simulink library "qss_tb_library"  (Simulink 6.3)
undefined symbols (not defined in the file): c_BT_E1, c_BT_E2, c_BT_E3, c_BT_E4, c_BT_L1, c_BT_L2, c_BT_L3, c_BT_L4, cc_done, delta_h_C_air, dw_GG_c, eta_EG_map, eta_EM_map, g, h, H_o_m, H_u, I_BT_max, i_FC_in, i_FC_max, k1, k2, k3, k4, k_cs, M_air, manual_gearbox, P_CVT_opt, Q_BT_0, Q_BT_IC, Q_BT_min, Q_SC_IC, r_wheel, rho, rho_f, t_c, T_CE_max, T_EG_c, T_EG_max, T_EM_max, U_BT_0, V_CE_map, V_FC_out, w_CE_max, w_CE_upper, w_CVT_opt, w_EG_row, w_EG_upper, w_EM_row, w_EM_upper, w_GG_c
(part 1 of 2)
settings Model: Creator=buehli  LastModifiedBy=mo  ExtModeAutoUpdateStatusClock=off

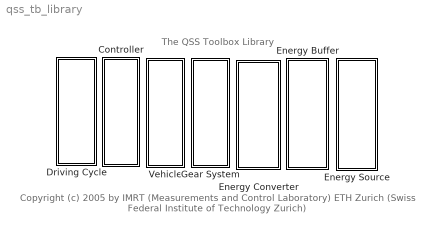
== system qss_tb_library ==
  note: Copyright (c) 2005 by IMRT (Measurements and Control Laboratory)
      | ETH Zurich (Swiss Federal Institute of Technology Zurich)
  note: The QSS Toolbox Library
  Controller : Subsystem  Orientation=up
      mask Display: disp('Controller')
  Driving Cycle : Subsystem  Orientation=up
      mask Display: disp('Driving Cycle')
  Energy Buffer : Subsystem  Orientation=up
      mask Display: disp('Energy Buffer')
  Energy Converter : Subsystem  Orientation=up
      mask Display: disp('Energy Converter')
  Energy Source : Subsystem  Orientation=up
      mask Display: disp('Energy Source')
  Gear System : Subsystem  Orientation=up
      mask Display: disp('Gear System')
  Vehicle : Subsystem  Orientation=up
      mask Display: disp('Vehicle')

== system qss_tb_library/Controller ==
  Battery Controller : Subsystem  AncestorBlock=qss_tb_library/Controller/Battery Controller  mask(Battery Controller){}
      mask help:
      | Control strategy (very primitive):
      | ========================
      | As soon as battery charge drops below level Q_BT_min, the CE/Generator
      | are started and operated at given load/speed for a fixed time period.
      | This time has been selected to guarantee the same battery level at the
      | end of the cycle.
      mask init:
      | init_BT_ctrl;
  CVT Controller : Subsystem  Tag=cvt controller  mask(CVT Controller){j_CVT_min=3, j_CVT_max=15, w_wheel_min=3, w_CVT_idle=100, w_CVT_upper=300}
      mask prompts: j_CVT_min "Lower gear ratio limit [-]"; j_CVT_max "Upper gear ratio limit [-]"; w_wheel_min "Minimum wheel speed [rad/s]"; w_CVT_idle "CVT idle speed [rad/s]"; w_CVT_upper "Maximum CVT speed [rad/s]"
      mask help:
      | This block calculates the optimum gear ratio and its change during one integration step for a CVT.
      |
      | Input:
      | =====
      | 	v		Speed [m/s]
      | 	dv		Acceleration [m/s^2]
      |
      | Output:
      | ======
      | 	v_delay		Speed one step delayed [m/s]
      | 	dv_delay	Acceleration one step delayed [m/s^2]
      | 	j_CVT		Gear ratio [-]
      | 	dj_CVT		Change of gear ratio [1/s]
      mask init:
      | init_CVT_ctrl;
  Control Unit (empty template) : Subsystem  Tag=control unit
      mask Type: Control Unit
      mask Description:
      | This block gives the user the opportunity to design his/her own control unit.
      | 
      | The user can define the inputs and outputs  by himself/herself.

== system qss_tb_library/Driving Cycle ==
  Driving Cycle : Subsystem  Tag=cycle  mask(Driving Cycle){cyclenr=Europe: NEDC, stepsize=1, autostop=on}
      mask prompts: cyclenr "Choose a cycle"; stepsize "Step size [s]"; autostop "Enable automatic simulation stop"
      mask help:
      | This block loads the cycle data such as time, speed, acceleration and gear number,  from the specified data file and makes it available on the output of the cycle block.
      |
      | Output:
      | ======
      | 	v	Speed [m/s]
      | 	dv	Acceleration [m/s^2]
      | 	i	Gear number [-]
      | 	x_tot	Total distance [m]
      |
      | Tip:
      | ===
      | Probably you don't need the gear number "i". If so you can terminate
      | it with a "Terminator" out of the "Simulink Library/Connections."
      |
      | Step size:
      | ========
      | Default value is 1. Don't change it, unless you are familiar with the programs of the QSS TB.
      |
      | Enable automatic simulation stop:
      | ===========================
      | Stops the simulation automatically at the end of the cycle.
      | Be careful: If you have a component in your model that has to run after the cycle has finished, e.g. a battery to charge, remove the mark!
      mask init:
      | init_driving_cycle;
      mask StyleString: popup(Europe: ECE manual|Europe: ECE R15 spez|Europe: ECE R15|Europe: EUDC|Europe: EUDC manual|Europe: City|Europe: City manual|Europe: NEDC|Europe: NEDC manual|Japan:  10-15-Mode|Japan:  10-Mode|Japan:  10-Mode-3|Japan:  11-Mode|Japan:  11-Mode-4|Japan:  15-Mode|USA:    City-I|USA:    City-II|USA:    FTP-75|USA:    FTP-Highway),edit,checkbox
      mask Display: plot(T_zplot, V_zplot);

== system qss_tb_library/Energy Buffer ==
  Battery : Subsystem  Tag=battery  mask(Battery){I_0=100, Q_BT_IC_rel=27.78, t_ch=20}
      mask prompts: I_0 "Energy capacity of battery [Ah]"; Q_BT_IC_rel "Initial charge of battery [%]"; t_ch "Current limit: minimum time to charge/discharge the battery [min]"
      mask help:
      | This block simulates a battery.
      | The resistance depends on the charge state and the charge/discharge current of the battery. The battery has an open circuit voltage of 130 V (fully charged).
      |
      | Input:
      | =====
      | 	x_tot	Total distance [m]
      | 	P_BT	Power from/to the battery [W]
      | 		P_BT < 0: battery charging
      | 		P_BT > 0: battery discharging
      |
      | Output:
      | ======
      | 	Q_BT	Current charge of the battery [C]
      | 	V_BT	Energy consumption [kWh/100 km]
      mask init:
      | init_BT;
  Supercapacitor : Subsystem  Tag=supercap  mask(Supercapacitor){C_SC=8, R_SC=0.72, U_SC_max=225, P_SC_max=17500, Q_SC_IC_rel=95, N_SC=6}
      mask prompts: C_SC "Capacity of each supercap [F]"; R_SC "Internal resistance of each supercap [Ohm]"; U_SC_max "Maximum voltage of each supercap  [V]"; P_SC_max "Maximum power of each supercap [W]"; Q_SC_IC_rel "Initial charge of each supercap [%]"; N_SC "Number of supercaps (parallel connection) [-]"
      mask help:
      | The supercap is a fast electric energy buffer.
      |
      | Input:
      | =====
      | 	P_SC	Power to/from the supercap [W]
      | 		P_SC < 0: SC charging
      | 		P_SC > 0: SC discharging
      |
      | Output:
      | ======
      | 	U_SC	Voltage of the supercap [V]
      mask init:
      | init_SC;

== system qss_tb_library/Energy Converter ==
  Combustion Engine (Willans-approximation) : Subsystem  Tag=combustion engine  AncestorBlock=qss_lib/Energy Converter/combustion engine  mask(Combustion Engine (based on Willans approximation)){engine_type=Otto, V_d=0.708, theta_CE=0.05, S=50, B=45, w_CE_idle=105, P_CE_idle=2600, P_aux=300, e=0.46, PI=2, p_me0g=1, ENABLE_FUEL_CUTOFF=on, T_CE_cutoff=5, P_CE_cutoff=0}
      mask prompts: engine_type "Engine type"; V_d "Displacement [l]"; theta_CE "Engine inertia [kg*m^2]"; S "Stroke [mm]"; B "Bore diameter [mm]"; w_CE_idle "Engine speed at idle [rad/s]"; P_CE_idle "Engine power at idle [W]"; P_aux "Power required by auxiliaries  [W]"; e "1. Willans parameter: Engine internal thermodynamic efficiency [-]"; PI "2. Willans parameter: Maximum boost ratio [-]"; p_me0g "3. Willans parameter: Gas exchange losses [bar]"; ENABLE_FUEL_CUTOFF "Enable fuel cutoff"; T_CE_cutoff "Engine torque at fuel cutoff [Nm]"; P_CE_cutoff "Power at fuel cutoff [W]"
      mask help:
      | This block simulates the behaviour of a combustion engine. The block is based on the Willans approximation with friction part based on the ETH model.
      |
      | Input:
      | =====
      | 	w_gear		Speed of the fly wheel [rad/s]
      | 	dw_gear	Acceleration of the fly wheel [rad/s^2]
      | 	T_gear		Torque on the fly wheel [Nm]
      |
      | Output:
      | ======
      | 	P_CE		Power produced by the combustion engine [W]
      mask init:
      | init_CE_willans;
      mask StyleString: popup(Otto|Diesel),edit,edit,edit,edit,edit,edit,edit,edit,edit,edit,checkbox,edit,edit
  Combustion Engine (consumption map) : Subsystem  Tag=combustion engine  AncestorBlock=QSS_TB_lib/Energy Converter/Combustion Engine  mask(Combustion Engine (based on consumption map)){engine_type=Otto, V_d=0.708, scale_CE=1, theta_CE=0.05, w_CE_idle=105, P_CE_idle=2600, P_aux=300, ENABLE_FUEL_CUTOFF=on, T_CE_cutoff=5, P_CE_cutoff=0}
      mask prompts: engine_type "Engine type"; V_d "Displacement [l]"; scale_CE "Engine scaling factor [-]"; theta_CE "Engine inertia [kg*m^2]"; w_CE_idle "Engine speed at idle [rad/s]"; P_CE_idle "Engine power at idle [W]"; P_aux "Power required by auxiliaries [W]"; ENABLE_FUEL_CUTOFF "Enable fuel cutoff"; T_CE_cutoff "Engine torque at fuel cutoff [Nm]"; P_CE_cutoff "Power at fuel cutoff [W]"
      mask help:
      | This block simulates the behaviour of a combustion engine. The block is based on a consumption map.
      |
      | Input:
      | =====
      | 	w_gear		Speed of the fly wheel [rad/s]
      | 	dw_gear	Acceleration of the fly wheel [rad/s^2]
      | 	T_gear		Torque on the fly wheel [Nm]
      |
      | Output:
      | ======
      | 	P_CE		Power produced by the combustion engine [W]
      mask init:
      | init_CE_map;
      mask StyleString: popup(Otto|Diesel),edit,edit,edit,edit,edit,edit,checkbox,edit,edit
  Electric Generator : Subsystem  AncestorBlock=QSS_TB_lib/Energy Converter/Electric Motor  mask(Electric Generator){scale_EG=1}
      mask prompts: scale_EG "Generator scaling factor [-]"
      mask help:
      | This block simulates the behaviour of an electric generator. The block is based on an efficiency map.
      |
      | Input:
      | =====
      | 	w_gear		Speed of the fly wheel [rad/s]
      | 	T_gear		Torque on the fly wheel [Nm]
      |
      | Output:
      | ======
      | 	P_EG		Power of the electric generator [W]
      mask init:
      | init_EG;
  Electric Motor : Subsystem  mask(Electric Motor){scale_EM=1, theta_EM=0.1, P_aux=0}
      mask prompts: scale_EM "Motor scaling factor [-]"; theta_EM "Motor inertia [kg*m2]"; P_aux "Power required by auxiliaries [W]"
      mask help:
      | This block simulates the behaviour of an electric motor. The block is based on an efficiency map.
      |
      | Input:
      | =====
      | 	w_gear		Speed of the fly wheel [rad/s]
      | 	dw_gear	Acceleration of the fly wheel [rad/s^2]
      | 	T_gear		Torque on the fly wheel [Nm]
      |
      | Output:
      | ======
      | 	P_EM		Power produced by the electric motor [W]
      mask init:
      | init_EM;
  Fuel Cell : Subsystem  Tag=fuelcell  mask(Fuel Cell){N_FC=880, A_FC=190 * 1e4, V_th=1.2, P_FC_idle=2000, eta_EM_C=0.75, eta_C=0.7, pi_C=1.3, T_air=25, l_air=1.5}
      mask prompts: N_FC "Number of fuel cells per stack (series connection) [-]"; A_FC "Size of fuel cell [m^2]"; V_th "Theoretical fuel cell voltage [V]"; P_FC_idle "Idle power [W]"; eta_EM_C "E-motor for air compressor efficiency [-]"; eta_C "Air compressor efficiency [-]"; pi_C "Air compression ratio [-]"; T_air "Air temperature [°C]"; l_air "Air to fuel ratio [-]"
      mask help:
      | This block simulates a fuel cell and converts fuel into electric energy.
      |
      | Input:
      | =====
      | 	P_in		Power required by the fuel cell [W]
      |
      | Output:
      | ======
      | 	P_FC		Power produced by the fuel cell [W]
      mask init:
      | init_FC;

== system qss_tb_library/Energy Source ==
  Display : Display
  Tank : Subsystem  Tag=tank  mask(Tank){fuel=Gasoline, flag_cold_start=on}
      mask prompts: flag_cold_start "Include cold start losses"
      mask help:
      | This block integrates the power (the fuel mass flow) required by the combustion engine or the fuel cell and calculates the energy consumption in liter/100 km.
      |
      | Input:
      | =====
      | 	P_fuel	Power (fuel mass flow) required [W]
      | 	x_tot	Total distance [m]
      |
      | Output:
      | ======
      | 	V	Fuel consumption [liter/100 km]
      mask init:
      | init_tank;
      mask StyleString: popup(Gasoline|Diesel|Hydrogen),checkbox
  wires:
  Tank/1(liter/100 km) -> Display/1

== system qss_tb_library/Gear System ==
  Continuously Variable Transmission : Subsystem  Tag=cvt  mask(CVT){e_CVT=0.97, P_CVT0=400, w_wheel_min=3}
      mask prompts: e_CVT "Efficiency [-]"; P_CVT0 "Idling losses (friction) [W]"; w_wheel_min "Minimum wheel speed beyond which losses are generated [rad/s]"
      mask help:
      | This block simulates a CVT transmission.
      |
      | Input:
      | =====
      | 	w_wheel	Speed of the wheel [rad/s]
      | 	dw_wheel	Acceleration of the wheel [rad/s^2],
      | 	T_wheel	Torque on the wheel [Nm]
      | 	j_CVT		Gear ratio [-]
      | 	dj_CVT		Change of gear ratio [1/s]
      |
      | Output:
      | ======
      | 	w_CVT		Speed of the fly wheel [rad/s]
      | 	dw_CVT	Acceleration of the fly wheel [rad/s^2]
      | 	T_CVT		Torque on the fly wheel [Nm]
      mask init:
      | init_CVT;
  Manual Gear Box : Subsystem  Tag=transmission  mask(Manual Gear Box){i_1=15.174, i_2=8.338, i_3=5.378, i_4=3.937, i_5=2.748, i_diff=1, e_GT=0.98, P_GT0=300, w_wheel_min=1}
      mask prompts: i_1 "1. gear [-]"; i_2 "2. gear [-]"; i_3 "3. gear [-]"; i_4 "4. gear [-]"; i_5 "5. gear [-]"; i_diff "Differential gear [-]"; e_GT "Efficiency [-]"; P_GT0 "Idling losses (friction) [W]"; w_wheel_min "Minimum wheel speed beyond which losses are generated [rad/s]"
      mask help:
      | This block simulates a manual gear box.
      |
      | Input:
      | =====
      | 	w_wheel	Speed of the wheel [rad/s]
      | 	dw_wheel	Acceleration of the wheel [rad/s^2],
      | 	T_wheel	Torque on the wheel [Nm]
      | 	i		Gear number [-]
      |
      | Output:
      | ======
      | 	w_MGB		Speed of the fly wheel [rad/s]
      | 	dw_MGB	Acceleration of the fly wheel [rad/s^2]
      | 	T_MGB		Torque on the fly wheel [Nm]
      mask init:
      | init_MGB;
  Simple Transmission : Subsystem  Tag=simple transmission  mask(Simple Transmission){gear_ratio=3, e_GT=0.98, P_GT0=50, w_wheel_min=1}
      mask prompts: gear_ratio "Gear ratio [-]"; e_GT "Efficiency [-]"; P_GT0 "Idling losses (friction) [W]"; w_wheel_min "Minimum wheel speed beyond which losses are generated [rad/s]"
      mask help:
      | This block simulates a transmission with a fixed gear ratio.
      |
      | Input:
      | =====
      | 	w_wheel	Speed of the wheel [rad/s]
      | 	dw_wheel	Acceleration of the wheel [rad/s^2]
      | 	T_wheel	Torque on the wheel [Nm]
      |
      | Output:
      | ======
      | 	w_trans		Speed of the fly wheel [rad/s]
      | 	dw_trans	Acceleration of the fly wheel [rad/s^2]
      | 	T_trans		Torque on the fly wheel [Nm]
      mask init:
      | init_transmission;

== system qss_tb_library/Vehicle ==
  Vehicle : Subsystem  Tag=vehicle  mask(Vehicle){m_f=750, mt2m_f=5, A_f=1.8, d_wheel=0.5, cw=0.22, mu=0.008}
      mask prompts: m_f "Total mass of the vehicle [kg]"; mt2m_f "Rotating mass [%]"; A_f "Vehicle cross section [m^2]"; d_wheel "Wheel diameter [m]"; cw "Drag coefficient [-]"; mu "Rolling friction coefficient [-]"
      mask help:
      | This block computes the power required from the vehicle.
      |
      | Input:
      | =====
      | 	v		Speed [m/s]
      | 	dv		Acceleration [m/s^2]
      |
      | Output:
      | ======
      | 	w_wheel	Speed of the wheel [rad/s]
      | 	dw_wheel	Acceleration of the wheel [rad/s^2]
      | 	T_wheel	Torque on the wheel [Nm]
      mask init:
      | init_vehicle;

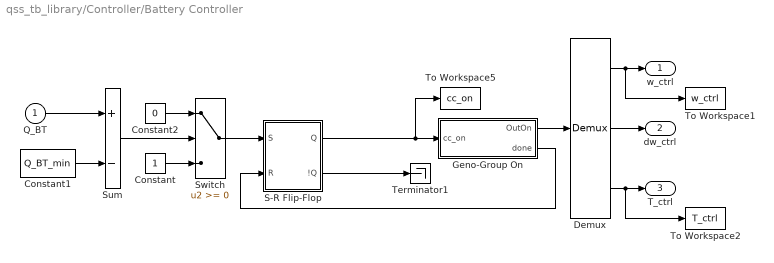
== system qss_tb_library/Controller/Battery Controller ==
  Q_BT : Inport
  Constant : Constant  OutDataTypeMode=boolean
  Constant1 : Constant  Value=Q_BT_min
  Constant2 : Constant  Value=0  OutDataTypeMode=boolean
  Demux : Demux  Outputs=3
  Geno-Group On : Subsystem
  S-R Flip-Flop : Subsystem
  Sum : Sum  Inputs=+-  SaturateOnIntegerOverflow=on  InputSameDT=on
  Switch : Switch  SaturateOnIntegerOverflow=on  InputSameDT=on
  Terminator1 : Terminator
  To Workspace1 : ToWorkspace  VariableName=w_ctrl  SampleTime=-1  SaveFormat=Array
  To Workspace2 : ToWorkspace  VariableName=T_ctrl  SampleTime=-1  SaveFormat=Array
  To Workspace5 : ToWorkspace  VariableName=cc_on  SampleTime=-1  SaveFormat=Array
  w_ctrl : Outport  InitialOutput=0
  dw_ctrl : Outport  Port=2  InitialOutput=0
  T_ctrl : Outport  Port=3  InitialOutput=0
  wires:
  S-R Flip-Flop/1(Q) -> To Workspace5/1, Geno-Group On/1(cc_on)
  Switch/1 -> S-R Flip-Flop/1(S)
  S-R Flip-Flop/2(!Q) -> Terminator1/1
  Geno-Group On/1(OutOn) -> Demux/1
  Demux/3 -> To Workspace2/1, T_ctrl/1
  Demux/2 -> dw_ctrl/1
  Demux/1 -> To Workspace1/1, w_ctrl/1
  Geno-Group On/2(done) -> S-R Flip-Flop/2(R)
  Q_BT/1 -> Sum/1
  Sum/1 -> Switch/2
  Constant2/1 -> Switch/1
  Constant/1 -> Switch/3
  Constant1/1 -> Sum/2

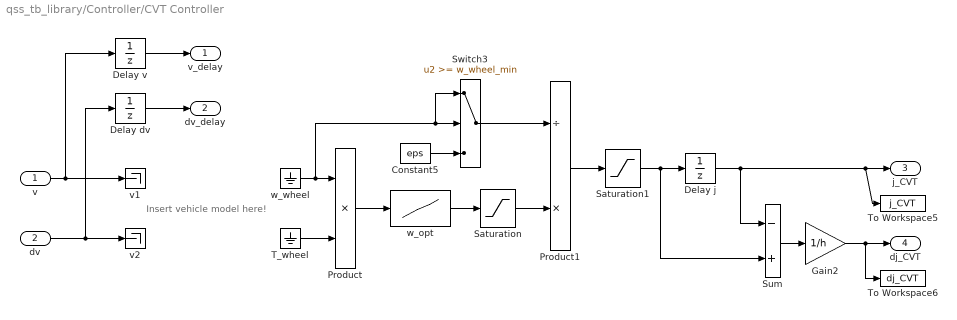
== system qss_tb_library/Controller/CVT Controller ==
  note: Insert vehicle
      | model here!
  v : Inport
  dv : Inport  Port=2
  Constant5 : Constant  Value=eps
  Delay dv : UnitDelay  SampleTime=h
  Delay j : UnitDelay  X0=j_CVT_min  SampleTime=h
  Delay v : UnitDelay  SampleTime=h
  Gain2 : Gain  Gain=1/h  SaturateOnIntegerOverflow=on
  Product : Product  SaturateOnIntegerOverflow=on  RndMeth=Zero  InputSameDT=on
  Product1 : Product  Inputs=/*  SaturateOnIntegerOverflow=on  RndMeth=Zero  InputSameDT=on
  Saturation : Saturate  UpperLimit=w_CVT_upper  LowerLimit=w_CVT_idle
  Saturation1 : Saturate  UpperLimit=j_CVT_max  LowerLimit=j_CVT_min
  Sum : Sum  Inputs=-+  SaturateOnIntegerOverflow=on  InputSameDT=on
  Switch3 : Switch  Threshold=w_wheel_min  SaturateOnIntegerOverflow=on  InputSameDT=on
  T_wheel : Ground
  To Workspace5 : ToWorkspace  VariableName=j_CVT  SampleTime=-1  SaveFormat=Array
  To Workspace6 : ToWorkspace  VariableName=dj_CVT  SampleTime=-1  SaveFormat=Array
  v1 : Terminator
  v2 : Terminator
  w_opt : Lookup  InputValues=P_CVT_opt  OutputValues=w_CVT_opt  SaturateOnIntegerOverflow=on
  w_wheel : Ground
  v_delay : Outport  InitialOutput=0
  dv_delay : Outport  Port=2  InitialOutput=0
  j_CVT : Outport  Port=3  InitialOutput=0
  dj_CVT : Outport  Port=4  InitialOutput=0
  wires:
  Gain2/1 -> To Workspace6/1, dj_CVT/1
  T_wheel/1 -> Product/2
  Product1/1 -> Saturation1/1
  Saturation/1 -> Product1/2
  w_wheel/1 -> Switch3/2, Switch3/1, Product/1
  Constant5/1 -> Switch3/3
  dv/1 -> Delay dv/1, v2/1
  v/1 -> Delay v/1, v1/1
  Delay dv/1 -> dv_delay/1
  Switch3/1 -> Product1/1
  Delay j/1 -> To Workspace5/1, j_CVT/1, Sum/1
  Saturation1/1 -> Delay j/1, Sum/2
  Product/1 -> w_opt/1
  w_opt/1 -> Saturation/1
  Delay v/1 -> v_delay/1
  Sum/1 -> Gain2/1

== system qss_tb_library/Controller/Control Unit (empty template) ==
  note: Control Unit: custom designed
  y 1 : Inport
  y p : Inport  Port=2
  Ground : Ground
  Ground1 : Ground
  Terminator : Terminator
  Terminator1 : Terminator
  u 1 : Outport  InitialOutput=0
  u m : Outport  Port=2  InitialOutput=0
  wires:
  Ground/1 -> u 1/1
  Ground1/1 -> u m/1
  y 1/1 -> Terminator/1
  y p/1 -> Terminator1/1

== system qss_tb_library/Driving Cycle/Driving Cycle ==
  note: Speed
  Clock : Clock
      settings: Decimation=10
  Cycle data : FromWorkspace  VariableName=[T_z, V_z, D_z, G_z]  SampleTime=h
  Demux : Demux  Outputs=3
  Differentiation : Subsystem
  Integration : Subsystem
  Terminator : Terminator
  Time : Display
  To Workspace1 : ToWorkspace  VariableName=t  SampleTime=-1  SaveFormat=Array
  To Workspace2 : ToWorkspace  VariableName=x_tot  SampleTime=-1  SaveFormat=Array
  To Workspace4 : ToWorkspace  VariableName=dv  SampleTime=-1  SaveFormat=Array
  To Workspace5 : ToWorkspace  VariableName=v  SampleTime=-1  SaveFormat=Array
  To Workspace6 : ToWorkspace  VariableName=i  SampleTime=-1  SaveFormat=Array
  v : Outport  InitialOutput=0
  dv : Outport  Port=2  InitialOutput=0
  i : Outport  Port=3  InitialOutput=0
  x_tot : Outport  Port=4  InitialOutput=0
  wires:
  Cycle data/1 -> Demux/1
  Differentiation/1(D_z) -> To Workspace4/1, dv/1
  Demux/2 -> Terminator/1
  Demux/1 -> Integration/1(V_z), v/1, To Workspace5/1, Differentiation/1(V_z)
  Integration/1(x_tot) -> x_tot/1, To Workspace2/1
  Demux/3 -> i/1, To Workspace6/1  "Gear ratio"
  Clock/1 -> Time/1, To Workspace1/1

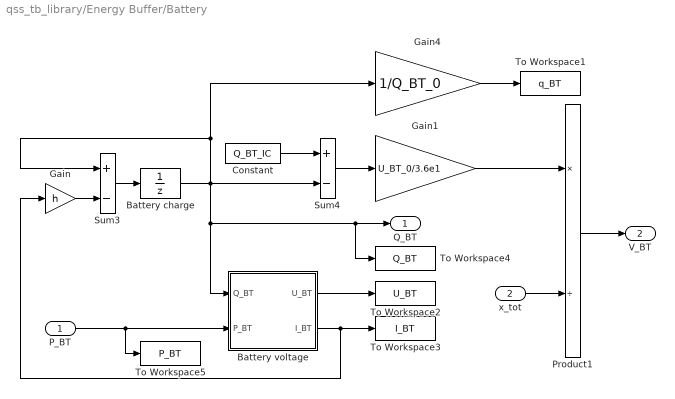
== system qss_tb_library/Energy Buffer/Battery ==
  P_BT : Inport
  x_tot : Inport  Port=2
  Battery charge : UnitDelay  X0=Q_BT_IC  SampleTime=h
  Battery voltage : Subsystem
  Constant : Constant  Value=Q_BT_IC
  Gain : Gain  Gain=h  SaturateOnIntegerOverflow=on
  Gain1 : Gain  Gain=U_BT_0/3.6e1  SaturateOnIntegerOverflow=on
  Gain4 : Gain  Gain=1/Q_BT_0  SaturateOnIntegerOverflow=on
  Product1 : Product  Inputs=*/  SaturateOnIntegerOverflow=on  RndMeth=Zero  InputSameDT=on
  Sum3 : Sum  Inputs=+-  SaturateOnIntegerOverflow=on  InputSameDT=on
  Sum4 : Sum  Inputs=+-  SaturateOnIntegerOverflow=on  InputSameDT=on
  To Workspace1 : ToWorkspace  VariableName=q_BT  SampleTime=-1  SaveFormat=Array
  To Workspace2 : ToWorkspace  VariableName=U_BT  SampleTime=-1  SaveFormat=Array
  To Workspace3 : ToWorkspace  VariableName=I_BT  SampleTime=-1  SaveFormat=Array
  To Workspace4 : ToWorkspace  VariableName=Q_BT  SampleTime=-1  SaveFormat=Array
  To Workspace5 : ToWorkspace  VariableName=P_BT  SampleTime=-1  SaveFormat=Array
  Q_BT : Outport  InitialOutput=0
  V_BT : Outport  Port=2  InitialOutput=0
  wires:
  Battery voltage/2(I_BT) -> Gain/1, To Workspace3/1
  Constant/1 -> Sum4/1
  Sum3/1 -> Battery charge/1
  Gain/1 -> Sum3/2
  Battery charge/1 -> Sum3/1, Gain4/1, Sum4/2, Battery voltage/1(Q_BT), Q_BT/1, To Workspace4/1
  Battery voltage/1(U_BT) -> To Workspace2/1
  x_tot/1 -> Product1/2
  Gain1/1 -> Product1/1
  Product1/1 -> V_BT/1
  Sum4/1 -> Gain1/1
  Gain4/1 -> To Workspace1/1
  P_BT/1 -> Battery voltage/2(P_BT), To Workspace5/1

== system qss_tb_library/Energy Buffer/Supercapacitor ==
  P_SC : Inport
  Fcn : Fcn  Expr=(-u[2]/C_SC+sqrt(u[2]^2/C_SC^2-4*R_SC*u[1]))/(2*R_SC)
  Gain : Gain  Gain=1/C_SC  SaturateOnIntegerOverflow=on
  Gain1 : Gain  Orientation=left  Gain=h  SaturateOnIntegerOverflow=on
  Mux : Mux  Inputs=2
  SC charge : UnitDelay  Orientation=left  X0=Q_SC_IC  SampleTime=h
  Sum3 : Sum  Orientation=left  SaturateOnIntegerOverflow=on  InputSameDT=on
  Supervision supercap : Subsystem
  To Workspace1 : ToWorkspace  VariableName=I_SC  SampleTime=1  SaveFormat=Array
  To Workspace2 : ToWorkspace  VariableName=U_SC  SampleTime=1  SaveFormat=Array
  To Workspace3 : ToWorkspace  VariableName=Q_SC  SampleTime=1  SaveFormat=Array
  To Workspace4 : ToWorkspace  VariableName=P_SC  SampleTime=1  SaveFormat=Array
  U_SC : Outport  InitialOutput=0
  wires:
  P_SC/1 -> Supervision supercap/2(P_SC), Mux/1, To Workspace4/1
  Gain/1 -> To Workspace2/1, U_SC/1
  Fcn/1 -> To Workspace1/1, Gain1/1
  SC charge/1 -> To Workspace3/1, Supervision supercap/1(Q_SC), Mux/2, Gain/1, Sum3/2
  Sum3/1 -> SC charge/1
  Mux/1 -> Fcn/1
  Gain1/1 -> Sum3/1

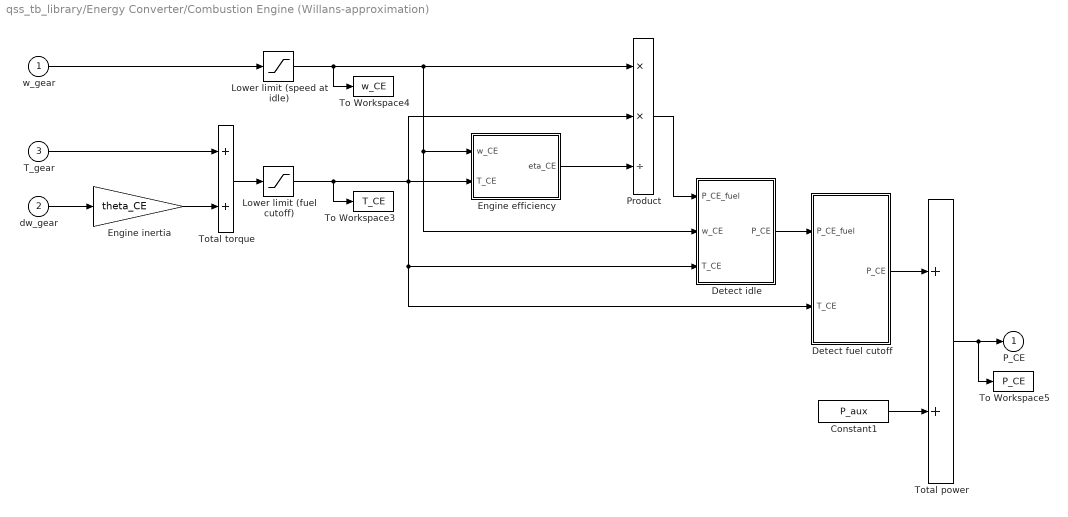
== system qss_tb_library/Energy Converter/Combustion Engine (Willans-approximation) ==
  w_gear : Inport
  dw_gear : Inport  Port=2
  T_gear : Inport  Port=3
  Constant1 : Constant  Value=P_aux
  Detect fuel cutoff : Subsystem  AncestorBlock=|
      | qss_tb_library/Energy Converter/Combustion Engine
      | (consumption map)/Detect fuel cutoff
  Detect idle : Subsystem
  Engine efficiency : Subsystem
  Engine inertia : Gain  Gain=theta_CE  SaturateOnIntegerOverflow=on
  Lower limit (fuel cutoff) : Saturate  UpperLimit=inf  LowerLimit=T_CE_cutoff
  Lower limit (speed at idle) : Saturate  UpperLimit=inf  LowerLimit=w_CE_idle
  Product : Product  Inputs=**/  SaturateOnIntegerOverflow=on  RndMeth=Zero  InputSameDT=on
  To Workspace3 : ToWorkspace  VariableName=T_CE  SampleTime=-1  SaveFormat=Array
  To Workspace4 : ToWorkspace  VariableName=w_CE  SampleTime=-1  SaveFormat=Array
  To Workspace5 : ToWorkspace  VariableName=P_CE  SampleTime=-1  SaveFormat=Array
  Total power : Sum  SaturateOnIntegerOverflow=on  InputSameDT=on
  Total torque : Sum  SaturateOnIntegerOverflow=on  InputSameDT=on
  P_CE : Outport  InitialOutput=0
  wires:
  Engine efficiency/1(eta_CE) -> Product/3
  T_gear/1 -> Total torque/1
  dw_gear/1 -> Engine inertia/1
  Total torque/1 -> Lower limit (fuel cutoff)/1
  Engine inertia/1 -> Total torque/2
  Lower limit (fuel cutoff)/1 -> Detect idle/3(T_CE), Detect fuel cutoff/2(T_CE), Engine efficiency/2(T_CE), Product/2, To Workspace3/1
  Lower limit (speed at idle)/1 -> To Workspace4/1, Engine efficiency/1(w_CE), Detect idle/2(w_CE), Product/1
  w_gear/1 -> Lower limit (speed at idle)/1
  Product/1 -> Detect idle/1(P_CE_fuel)
  Detect idle/1(P_CE) -> Detect fuel cutoff/1(P_CE_fuel)
  Detect fuel cutoff/1(P_CE) -> Total power/1
  Total power/1 -> P_CE/1, To Workspace5/1
  Constant1/1 -> Total power/2

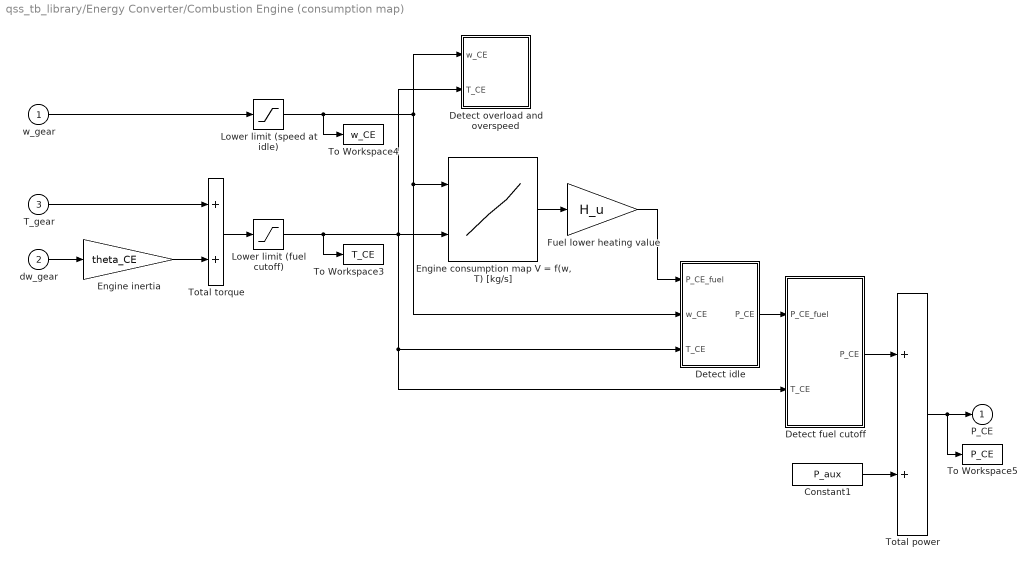
== system qss_tb_library/Energy Converter/Combustion Engine (consumption map) ==
  w_gear : Inport
  dw_gear : Inport  Port=2
  T_gear : Inport  Port=3
  Constant1 : Constant  Value=P_aux
  Detect fuel cutoff : Subsystem
  Detect idle : Subsystem
  Detect overload and overspeed : Subsystem
  "Engine consumption map V = f(w, T) [kg/s]" : Lookup2D  RowIndex=w_CE_row  ColumnIndex=T_CE_col  OutputValues=V_CE_map
  Engine inertia : Gain  Gain=theta_CE  SaturateOnIntegerOverflow=on
  Fuel lower heating value : Gain  Gain=H_u  SaturateOnIntegerOverflow=on
  Lower limit (fuel cutoff) : Saturate  UpperLimit=inf  LowerLimit=T_CE_cutoff
  Lower limit (speed at idle) : Saturate  UpperLimit=inf  LowerLimit=w_CE_idle
  To Workspace3 : ToWorkspace  VariableName=T_CE  SampleTime=-1  SaveFormat=Array
  To Workspace4 : ToWorkspace  VariableName=w_CE  SampleTime=-1  SaveFormat=Array
  To Workspace5 : ToWorkspace  VariableName=P_CE  SampleTime=-1  SaveFormat=Array
  Total power : Sum  SaturateOnIntegerOverflow=on  InputSameDT=on
  Total torque : Sum  SaturateOnIntegerOverflow=on  InputSameDT=on
  P_CE : Outport  InitialOutput=0
  wires:
  T_gear/1 -> Total torque/1
  dw_gear/1 -> Engine inertia/1
  Total torque/1 -> Lower limit (fuel cutoff)/1
  Engine inertia/1 -> Total torque/2
  Lower limit (speed at idle)/1 -> Detect overload and overspeed/1(w_CE), Detect idle/2(w_CE), "Engine consumption map V = f(w, T) [kg/s]"/1, To Workspace4/1
  w_gear/1 -> Lower limit (speed at idle)/1
  Fuel lower heating value/1 -> Detect idle/1(P_CE_fuel)
  Detect idle/1(P_CE) -> Detect fuel cutoff/1(P_CE_fuel)
  "Engine consumption map V = f(w, T) [kg/s]"/1 -> Fuel lower heating value/1
  Detect fuel cutoff/1(P_CE) -> Total power/1
  Total power/1 -> P_CE/1, To Workspace5/1
  Constant1/1 -> Total power/2
  Lower limit (fuel cutoff)/1 -> Detect overload and overspeed/2(T_CE), "Engine consumption map V = f(w, T) [kg/s]"/2, Detect idle/3(T_CE), Detect fuel cutoff/2(T_CE), To Workspace3/1

== system qss_tb_library/Energy Converter/Electric Generator ==
  w_gear : Inport
  T_gear : Inport  Port=2
  Detect overload and overspeed : Subsystem
  "Efficiency eta = f(w, T)" : Lookup2D  RowIndex=w_EG_row  ColumnIndex=T_EG_col  OutputValues=eta_EG_map
  Product : Product  Inputs=3  SaturateOnIntegerOverflow=on  RndMeth=Zero  InputSameDT=on
  To Workspace1 : ToWorkspace  VariableName=w_EG  SampleTime=-1  SaveFormat=Array
  To Workspace2 : ToWorkspace  VariableName=T_EG  SampleTime=-1  SaveFormat=Array
  To Workspace5 : ToWorkspace  VariableName=P_EG  SampleTime=-1  SaveFormat=Array
  P_EG : Outport  InitialOutput=0
  wires:
  T_gear/1 -> Product/2, "Efficiency eta = f(w, T)"/2, Detect overload and overspeed/2(T_EG), To Workspace2/1
  "Efficiency eta = f(w, T)"/1 -> Product/1
  Product/1 -> P_EG/1, To Workspace5/1
  w_gear/1 -> Product/3, "Efficiency eta = f(w, T)"/1, Detect overload and overspeed/1(w_EG), To Workspace1/1

== system qss_tb_library/Energy Converter/Electric Motor ==
  w_gear : Inport
  dw_gear : Inport  Port=2
  T_gear : Inport  Port=3
  Constant1 : Constant  Value=P_aux
  Detect overload and overspeed : Subsystem
  "Efficiency eta = f(w, T)" : Lookup2D  RowIndex=w_EM_row  ColumnIndex=T_EM_col  OutputValues=eta_EM_map
  Gain1 : Gain  Gain=theta_EM  SaturateOnIntegerOverflow=on
  Product : Product  Inputs=3  SaturateOnIntegerOverflow=on  RndMeth=Zero  InputSameDT=on
  To Workspace1 : ToWorkspace  VariableName=w_EM  SampleTime=-1  SaveFormat=Array
  To Workspace2 : ToWorkspace  VariableName=T_EM  SampleTime=-1  SaveFormat=Array
  To Workspace5 : ToWorkspace  VariableName=P_EM  SampleTime=-1  SaveFormat=Array
  Total power : Sum  SaturateOnIntegerOverflow=on  InputSameDT=on
  Total torque : Sum  SaturateOnIntegerOverflow=on  InputSameDT=on
  P_EM : Outport  InitialOutput=0
  wires:
  w_gear/1 -> Detect overload and overspeed/1(w_EM), "Efficiency eta = f(w, T)"/1, Product/3, To Workspace1/1
  "Efficiency eta = f(w, T)"/1 -> Product/1
  dw_gear/1 -> Gain1/1
  T_gear/1 -> Total torque/2
  Gain1/1 -> Total torque/1
  Total torque/1 -> Detect overload and overspeed/2(T_EM), "Efficiency eta = f(w, T)"/2, Product/2, To Workspace2/1
  Constant1/1 -> Total power/2
  Product/1 -> Total power/1
  Total power/1 -> P_EM/1, To Workspace5/1

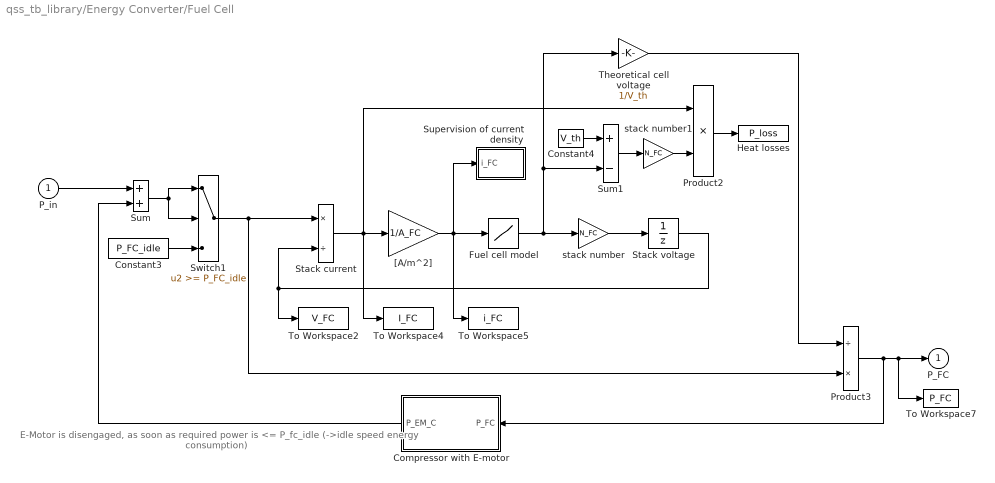
== system qss_tb_library/Energy Converter/Fuel Cell ==
  note: E-Motor is disengaged, as soon as required power
      |  is <= P_fc_idle (->idle speed energy consumption)
  P_in : Inport
  Compressor with E-motor : Subsystem  Orientation=left
  Constant3 : Constant  Value=P_FC_idle
  Constant4 : Constant  Value=V_th
  Fuel cell model : Lookup  InputValues=i_FC_in  OutputValues=V_FC_out  SaturateOnIntegerOverflow=on
  Heat losses : ToWorkspace  VariableName=P_loss  SampleTime=1  SaveFormat=Array
  Product2 : Product  SaturateOnIntegerOverflow=on  RndMeth=Zero  InputSameDT=on
  Product3 : Product  Inputs=/*  SaturateOnIntegerOverflow=on  RndMeth=Zero  InputSameDT=on
  Stack current : Product  Inputs=*/  SaturateOnIntegerOverflow=on  RndMeth=Zero  InputSameDT=on
  Stack voltage : UnitDelay  X0=10  SampleTime=h
  Sum : Sum  SaturateOnIntegerOverflow=on  InputSameDT=on
  Sum1 : Sum  Inputs=+-  SaturateOnIntegerOverflow=on  InputSameDT=on
  Supervision of current density : Subsystem
  Switch1 : Switch  Threshold=P_FC_idle  SaturateOnIntegerOverflow=on  InputSameDT=on
  Theoretical cell voltage : Gain  Gain=1/V_th  SaturateOnIntegerOverflow=on
  To Workspace2 : ToWorkspace  VariableName=V_FC  SampleTime=1  SaveFormat=Array
  To Workspace4 : ToWorkspace  VariableName=I_FC  SampleTime=1  SaveFormat=Array
  To Workspace5 : ToWorkspace  VariableName=i_FC  SampleTime=1  SaveFormat=Array
  To Workspace7 : ToWorkspace  VariableName=P_FC  SampleTime=1  SaveFormat=Array
  "[A/m^2]" : Gain  Gain=1/A_FC  SaturateOnIntegerOverflow=on
  stack number : Gain  Gain=N_FC  SaturateOnIntegerOverflow=on
  stack number1 : Gain  Gain=N_FC  SaturateOnIntegerOverflow=on
  P_FC : Outport  InitialOutput=0
  wires:
  Compressor with E-motor/1(P_EM_C) -> Sum/2
  Switch1/1 -> Stack current/1, Product3/2
  Constant3/1 -> Switch1/3
  Sum/1 -> Switch1/2, Switch1/1
  P_in/1 -> Sum/1
  Constant4/1 -> Sum1/1
  stack number/1 -> Stack voltage/1
  Sum1/1 -> stack number1/1
  stack number1/1 -> Product2/2
  "[A/m^2]"/1 -> Fuel cell model/1, To Workspace5/1, Supervision of current density/1("   i_FC")
  Theoretical cell voltage/1 -> Product3/1
  Fuel cell model/1 -> stack number/1, Sum1/2, Theoretical cell voltage/1
  Stack current/1 -> "[A/m^2]"/1, Product2/1, To Workspace4/1
  Stack voltage/1 -> Stack current/2, To Workspace2/1
  Product3/1 -> P_FC/1, To Workspace7/1, Compressor with E-motor/1(P_FC)
  Product2/1 -> Heat losses/1

== system qss_tb_library/Energy Source/Tank ==
  P_fuel : Inport
  x_tot : Inport  Port=2
  Factor for cold start : Gain  Gain=k_cs  SaturateOnIntegerOverflow=on
  Fu2131el density : Gain  Gain=1/rho_f  SaturateOnIntegerOverflow=on
  Gain3 : Gain  Gain=1e5  SaturateOnIntegerOverflow=on
  Integration : Subsystem
  Product : Product  Inputs=*/  SaturateOnIntegerOverflow=on  RndMeth=Zero  InputSameDT=on
  To Workspace7 : ToWorkspace  VariableName=V_liter  SampleTime=-1  SaveFormat=Array
  liter/100 km : Outport  InitialOutput=0
  wires:
  P_fuel/1 -> Integration/1(P_fuel)
  x_tot/1 -> Product/2
  Integration/1(m_fuel) -> Fu2131el density/1
  Gain3/1 -> liter/100 km/1, To Workspace7/1
  Fu2131el density/1 -> Product/1
  Product/1 -> Factor for cold start/1
  Factor for cold start/1 -> Gain3/1

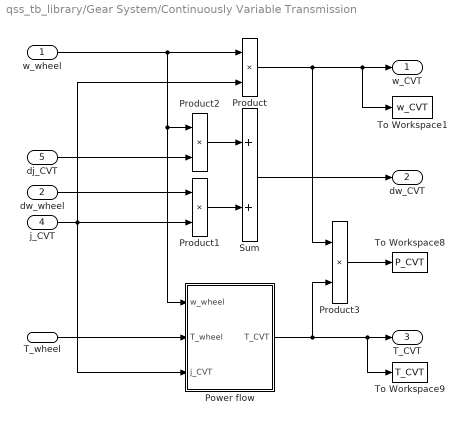
== system qss_tb_library/Gear System/Continuously Variable Transmission ==
  w_wheel : Inport
  dw_wheel : Inport  Port=2
  T_wheel : Inport  Port=3
  j_CVT : Inport  Port=4
  dj_CVT : Inport  Port=5
  Power flow : Subsystem
  Product{,1..3} (4 alike) : Product  SaturateOnIntegerOverflow=on  RndMeth=Zero  InputSameDT=on
  Sum : Sum  SaturateOnIntegerOverflow=on  InputSameDT=on
  To Workspace1 : ToWorkspace  VariableName=w_CVT  SampleTime=-1  SaveFormat=Array
  To Workspace8 : ToWorkspace  VariableName=P_CVT  SampleTime=-1  SaveFormat=Array
  To Workspace9 : ToWorkspace  VariableName=T_CVT  SampleTime=-1  SaveFormat=Array
  w_CVT : Outport  InitialOutput=0
  dw_CVT : Outport  Port=2  InitialOutput=0
  T_CVT : Outport  Port=3  InitialOutput=0
  wires:
  w_wheel/1 -> Power flow/1(w_wheel), Product2/1, Product/1
  Power flow/1(T_CVT) -> To Workspace9/1, T_CVT/1, Product3/2
  Product/1 -> Product3/1, w_CVT/1, To Workspace1/1
  Sum/1 -> dw_CVT/1
  dw_wheel/1 -> Product1/1
  dj_CVT/1 -> Product2/2
  j_CVT/1 -> Product1/2, Product/2, Power flow/3(j_CVT)
  Product1/1 -> Sum/2
  Product2/1 -> Sum/1
  T_wheel/1 -> Power flow/2(T_wheel)
  Product3/1 -> To Workspace8/1

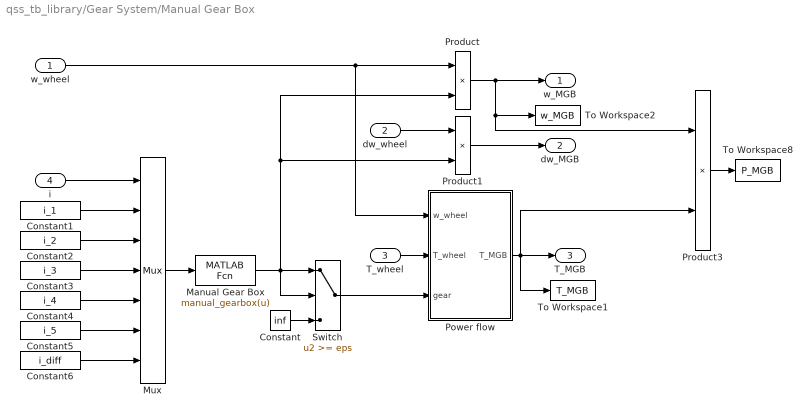
== system qss_tb_library/Gear System/Manual Gear Box ==
  w_wheel : Inport
  dw_wheel : Inport  Port=2
  T_wheel : Inport  Port=3
  i : Inport  Port=4
  Constant : Constant  Value=inf
  Constant1 : Constant  Value=i_1
  Constant2 : Constant  Value=i_2
  Constant3 : Constant  Value=i_3
  Constant4 : Constant  Value=i_4
  Constant5 : Constant  Value=i_5
  Constant6 : Constant  Value=i_diff
  Manual Gear Box : MATLABFcn  MATLABFcn=manual_gearbox(u)  OutputDimensions=1
  Mux : Mux  Inputs=7
  Power flow : Subsystem
  Product : Product  SaturateOnIntegerOverflow=on  RndMeth=Zero  InputSameDT=on
  Product1 : Product  SaturateOnIntegerOverflow=on  RndMeth=Zero  InputSameDT=on
  Product3 : Product  SaturateOnIntegerOverflow=on  RndMeth=Zero  InputSameDT=on
  Switch : Switch  Threshold=eps  SaturateOnIntegerOverflow=on  InputSameDT=on
  To Workspace1 : ToWorkspace  VariableName=T_MGB  SampleTime=-1  SaveFormat=Array
  To Workspace2 : ToWorkspace  VariableName=w_MGB  SampleTime=-1  SaveFormat=Array
  To Workspace8 : ToWorkspace  VariableName=P_MGB  SampleTime=-1  SaveFormat=Array
  w_MGB : Outport  InitialOutput=0
  dw_MGB : Outport  Port=2  InitialOutput=0
  T_MGB : Outport  Port=3  InitialOutput=0
  wires:
  Power flow/1(T_MGB) -> T_MGB/1, Product3/2, To Workspace1/1
  Product/1 -> w_MGB/1, Product3/1, To Workspace2/1
  Constant/1 -> Switch/3
  w_wheel/1 -> Product/1, Power flow/1(w_wheel)
  Product1/1 -> dw_MGB/1
  dw_wheel/1 -> Product1/1
  Manual Gear Box/1 -> Product/2, Product1/2, Switch/2, Switch/1
  Product3/1 -> To Workspace8/1
  Switch/1 -> Power flow/3(gear)
  T_wheel/1 -> Power flow/2(T_wheel)
  Constant1/1 -> Mux/2
  Constant2/1 -> Mux/3
  Constant3/1 -> Mux/4
  Constant4/1 -> Mux/5
  Constant5/1 -> Mux/6
  Constant6/1 -> Mux/7
  i/1 -> Mux/1
  Mux/1 -> Manual Gear Box/1

== system qss_tb_library/Gear System/Simple Transmission ==
  w_wheel : Inport
  dw_wheel : Inport  Port=2
  T_wheel : Inport  Port=3
  Constant : Constant  Value=gear_ratio
  Power flow : Subsystem
  Product : Product  SaturateOnIntegerOverflow=on  RndMeth=Zero  InputSameDT=on
  Product1 : Product  SaturateOnIntegerOverflow=on  RndMeth=Zero  InputSameDT=on
  Product3 : Product  SaturateOnIntegerOverflow=on  RndMeth=Zero  InputSameDT=on
  To Workspace1 : ToWorkspace  VariableName=w_trans  SampleTime=-1  SaveFormat=Array
  To Workspace2 : ToWorkspace  VariableName=T_trans  SampleTime=-1  SaveFormat=Array
  To Workspace3 : ToWorkspace  VariableName=P_trans  SampleTime=-1  SaveFormat=Array
  w_trans : Outport  InitialOutput=0
  dw_trans : Outport  Port=2  InitialOutput=0
  T_trans : Outport  Port=3  InitialOutput=0
  wires:
  Power flow/1(T_trans) -> T_trans/1, To Workspace2/1, Product3/2
  Product1/1 -> dw_trans/1
  Product/1 -> w_trans/1, To Workspace1/1, Product3/1
  dw_wheel/1 -> Product1/1
  T_wheel/1 -> Power flow/2(T_wheel)
  Constant/1 -> Power flow/3(gear_ratio), Product1/2, Product/2
  w_wheel/1 -> Product/1, Power flow/1(w_wheel)
  Product3/1 -> To Workspace3/1

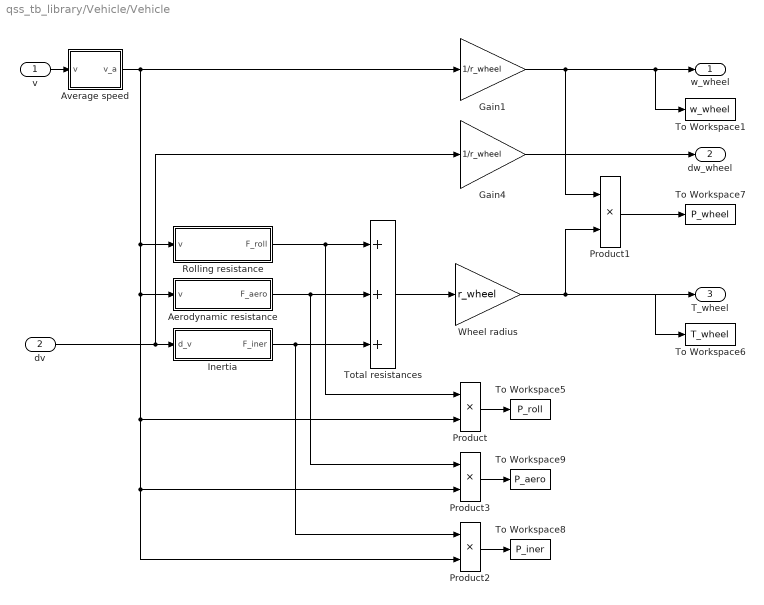
== system qss_tb_library/Vehicle/Vehicle ==
  v : Inport
  dv : Inport  Port=2
  Aerodynamic resistance : Subsystem
  Average speed : Subsystem
  Gain1 : Gain  Gain=1/r_wheel  SaturateOnIntegerOverflow=on
  Gain4 : Gain  Gain=1/r_wheel  SaturateOnIntegerOverflow=on
  Inertia : Subsystem
  Product{,1..3} (4 alike) : Product  SaturateOnIntegerOverflow=on  RndMeth=Zero  InputSameDT=on
  Rolling resistance : Subsystem
  To Workspace1 : ToWorkspace  VariableName=w_wheel  SampleTime=-1  SaveFormat=Array
  To Workspace5 : ToWorkspace  VariableName=P_roll  SampleTime=-1  SaveFormat=Array
  To Workspace6 : ToWorkspace  VariableName=T_wheel  SampleTime=-1  SaveFormat=Array
  To Workspace7 : ToWorkspace  VariableName=P_wheel  SampleTime=-1  SaveFormat=Array
  To Workspace8 : ToWorkspace  VariableName=P_iner  SampleTime=-1  SaveFormat=Array
  To Workspace9 : ToWorkspace  VariableName=P_aero  SampleTime=-1  SaveFormat=Array
  Total resistances : Sum  Inputs=+++  SaturateOnIntegerOverflow=on  InputSameDT=on
  Wheel radius : Gain  Gain=r_wheel  SaturateOnIntegerOverflow=on
  w_wheel : Outport  InitialOutput=0
  dw_wheel : Outport  Port=2  InitialOutput=0
  T_wheel : Outport  Port=3  InitialOutput=0
  wires:
  Gain4/1 -> dw_wheel/1
  Gain1/1 -> Product1/1, w_wheel/1, To Workspace1/1
  Rolling resistance/1(F_roll) -> Total resistances/1, Product/1
  Aerodynamic resistance/1(F_aero) -> Product3/1, Total resistances/2
  Inertia/1(F_iner) -> Total resistances/3, Product2/1
  Total resistances/1 -> Wheel radius/1
  Wheel radius/1 -> T_wheel/1, Product1/2, To Workspace6/1
  Average speed/1(v_a) -> Gain1/1, Aerodynamic resistance/1(v), Product/2, Product3/2, Product2/2, Rolling resistance/1(v)
  dv/1 -> Inertia/1(d_v), Gain4/1
  v/1 -> Average speed/1(v)
  Product2/1 -> To Workspace8/1
  Product3/1 -> To Workspace9/1
  Product1/1 -> To Workspace7/1
  Product/1 -> To Workspace5/1

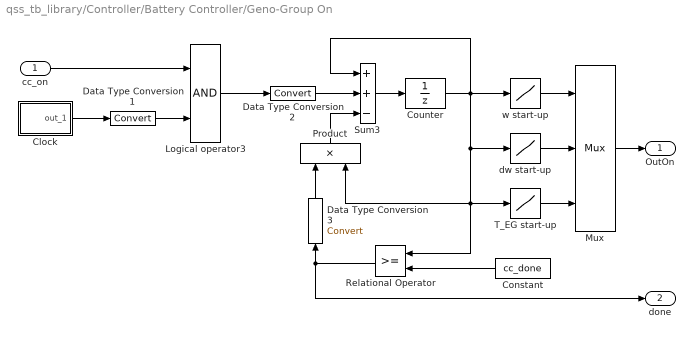
== system qss_tb_library/Controller/Battery Controller/Geno-Group On ==
  cc_on : Inport
  Clock : Subsystem  mask(Digital clock){@1=2}
      mask prompts: @1 "Period:"
      mask help:
      | Digital clock.
      | Output is set to 1 for the first half of the period.
      mask init:
      | duration = @1/2;
      mask Help: Digital clock for logic systems.
      mask Display: plot(0,0,100,100,[90,75,75,60,60,35,35,20,20,10],[20,20,80,80,19,20,80,80,20,20])
  Constant : Constant  Orientation=left  Value=cc_done
  Counter : UnitDelay  SampleTime=h
  Data Type Conversion1 : DataTypeConversion  OutDataTypeMode=boolean
  Data Type Conversion2 : DataTypeConversion  OutDataTypeMode=double
  Data Type Conversion3 : DataTypeConversion  Orientation=up  OutDataTypeMode=double
  Logical operator3 : Logic
  Mux : Mux  Inputs=3
  Product : Product  Orientation=up  SaturateOnIntegerOverflow=on  RndMeth=Zero  InputSameDT=on
  Relational Operator : RelationalOperator  Orientation=left  LogicOutDataTypeMode=Boolean  InputSameDT=on
  Sum3 : Sum  Inputs=++-  SaturateOnIntegerOverflow=on  InputSameDT=on
  T_EG start-up : Lookup  InputValues=t_c  OutputValues=T_EG_c  SaturateOnIntegerOverflow=on
  dw start-up : Lookup  InputValues=t_c  OutputValues=dw_GG_c  SaturateOnIntegerOverflow=on
  w start-up : Lookup  InputValues=t_c  OutputValues=w_GG_c  SaturateOnIntegerOverflow=on
  OutOn : Outport  InitialOutput=0
  done : Outport  Port=2  InitialOutput=0
  wires:
  Data Type Conversion3/1 -> Product/1
  Data Type Conversion2/1 -> Sum3/2
  Data Type Conversion1/1 -> Logical operator3/2
  Mux/1 -> OutOn/1
  T_EG start-up/1 -> Mux/3
  dw start-up/1 -> Mux/2
  w start-up/1 -> Mux/1
  Logical operator3/1 -> Data Type Conversion2/1
  Counter/1 -> Sum3/1, dw start-up/1, T_EG start-up/1, Product/2, Relational Operator/1, w start-up/1
  Sum3/1 -> Counter/1
  Clock/1(out_1) -> Data Type Conversion1/1
  cc_on/1 -> Logical operator3/1
  Product/1 -> Sum3/3
  Constant/1 -> Relational Operator/2
  Relational Operator/1 -> Data Type Conversion3/1, done/1

== system qss_tb_library/Controller/Battery Controller/S-R Flip-Flop ==
  S : Inport
  R : Inport  Port=2
  Demux : Demux  Outputs=2
  Logic : CombinatorialLogic  TruthTable=[0 1;0 1;1 0;0 1;1 0;0 1;1 0;1 0]
  Memory : Memory  Orientation=left  InheritSampleTime=on
  Mux : Mux  Inputs=3
  Q : Outport  InitialOutput=0
  !Q : Outport  Port=2  InitialOutput=1
  wires:
  R/1 -> Mux/3
  S/1 -> Mux/2
  Memory/1 -> Mux/1
  Demux/1 -> Memory/1, Q/1
  Demux/2 -> !Q/1
  Logic/1 -> Demux/1
  Mux/1 -> Logic/1

== system qss_tb_library/Driving Cycle/Driving Cycle/Differentiation ==
  V_z : Inport
  Sum1 : Sum  Inputs=+-  SaturateOnIntegerOverflow=on  InputSameDT=on
  Unit Delay1 : UnitDelay  SampleTime=h
  D_z : Outport  InitialOutput=0
  wires:
  Unit Delay1/1 -> Sum1/2
  V_z/1 -> Sum1/1, Unit Delay1/1
  Sum1/1 -> D_z/1

== system qss_tb_library/Driving Cycle/Driving Cycle/Integration ==
  V_z : Inport
  Gain4 : Gain  Gain=0.5*h  SaturateOnIntegerOverflow=on
  Plant : UnitDelay  X0=1  SampleTime=h
  Sum2 : Sum  SaturateOnIntegerOverflow=on  InputSameDT=on
  Sum4 : Sum  SaturateOnIntegerOverflow=on  InputSameDT=on
  Unit Delay2 : UnitDelay  SampleTime=h
  x_tot : Outport  InitialOutput=0
  wires:
  Sum2/1 -> Gain4/1
  Unit Delay2/1 -> Sum2/2
  V_z/1 -> Sum2/1, Unit Delay2/1
  Gain4/1 -> Sum4/2
  Sum4/1 -> Plant/1
  Plant/1 -> Sum4/1, x_tot/1

== system qss_tb_library/Energy Buffer/Battery/Battery voltage ==
  Q_BT : Inport
  P_BT : Inport  Port=2
  Charging : Subsystem
  Discharging : Subsystem
  Enable charging : Subsystem
  Enable discharging : Subsystem
  Enable idle : Subsystem
  Idle : Subsystem
  Product : Product  Inputs=/*  SaturateOnIntegerOverflow=on  RndMeth=Zero  InputSameDT=on
  Supervision battery : Subsystem
  Switch : Switch  Threshold=0.5  SaturateOnIntegerOverflow=on  InputSameDT=on
  Switch1 : Switch  Threshold=0.5  SaturateOnIntegerOverflow=on  InputSameDT=on
  U_BT : Outport  InitialOutput=0
  I_BT : Outport  Port=2  InitialOutput=0
  wires:
  Enable idle/1(e_Z) -> Idle/Enable
  Charging/1(U_BT_L) -> Switch/1
  Switch1/1 -> Switch/3
  Idle/1(U_BT_E) -> Switch1/3
  Discharging/1(U_BT_E) -> Switch1/1
  P_BT/1 -> Charging/2(P_BT), Enable charging/1(P_BT), Enable idle/1(P_BT), Product/2, Discharging/2(P_BT), Enable discharging/1(P_BT)
  Enable discharging/1(e_E) -> Discharging/Enable, Switch1/2
  Product/1 -> Supervision battery/3(I_BT), I_BT/1
  Q_BT/1 -> Supervision battery/1(Q_BT), Charging/1(Q_BT), Discharging/1(Q_BT), Idle/1(Q_BT)
  Enable charging/1(e_E) -> Charging/Enable, Switch/2
  Switch/1 -> Product/1, Supervision battery/2(U_BT), U_BT/1

== system qss_tb_library/Energy Buffer/Supercapacitor/Supervision supercap ==
  Q_SC : Inport
  P_SC : Inport  Port=2
  Charge: P > 0 : Gain  Gain=4*C_SC^2*R_SC  SaturateOnIntegerOverflow=on
  Constant6 : Constant  Value=U_SC_max
  Constant7 : Constant  Value=P_SC_max
  Gain : Gain  Gain=1/C_SC  SaturateOnIntegerOverflow=on
  Math Function : Math  Operator=square  SaturateOnIntegerOverflow=on
  Saturation1 : Saturate  UpperLimit=0  LowerLimit=-inf
  Saturation2 : Saturate  UpperLimit=0  LowerLimit=-inf
  Saturation3 : Saturate  UpperLimit=0  LowerLimit=-inf
  Stop Simulation : Stop
  Stop Simulation1 : Stop
  Stop Simulation2 : Stop
  Sum1 : Sum  Inputs=-+  SaturateOnIntegerOverflow=on  InputSameDT=on
  Sum2 : Sum  Inputs=+-  SaturateOnIntegerOverflow=on  InputSameDT=on
  Sum4 : Sum  SaturateOnIntegerOverflow=on  InputSameDT=on
  wires:
  Math Function/1 -> Sum2/1
  Q_SC/1 -> Math Function/1, Gain/1
  Constant7/1 -> Sum4/2
  Constant6/1 -> Sum1/2
  Sum4/1 -> Saturation3/1
  Sum2/1 -> Saturation2/1
  Gain/1 -> Sum1/1
  Sum1/1 -> Saturation1/1
  Charge: P > 0/1 -> Sum2/2
  P_SC/1 -> Charge: P > 0/1, Sum4/1
  Saturation1/1 -> Stop Simulation/1
  Saturation2/1 -> Stop Simulation1/1
  Saturation3/1 -> Stop Simulation2/1

== system qss_tb_library/Energy Converter/Combustion Engine (Willans-approximation)/Detect fuel cutoff ==
  P_CE_fuel : Inport
  T_CE : Inport  Port=2
  Constant1 : Constant  Value=ENABLE_FUEL_CUTOFF
  Constant3 : Constant  Value=P_CE_cutoff
  Decision : Switch  Threshold=0.5
  Detect fuel cutoff : Switch  Threshold=T_CE_cutoff + 0.01  SaturateOnIntegerOverflow=on  InputSameDT=on
  P_CE : Outport
  wires:
  Decision/1 -> P_CE/1
  Constant1/1 -> Decision/2
  Detect fuel cutoff/1 -> Decision/1
  P_CE_fuel/1 -> Decision/3, Detect fuel cutoff/1
  T_CE/1 -> Detect fuel cutoff/2
  Constant3/1 -> Detect fuel cutoff/3

== system qss_tb_library/Energy Converter/Combustion Engine (Willans-approximation)/Detect idle ==
  P_CE_fuel : Inport
  w_CE : Inport  Port=2
  T_CE : Inport  Port=3
  Constant3 : Constant  Value=P_CE_idle
  Idle detection : Fcn  Expr=(u(1) <= w_CE_idle) * (u(2) <= T_CE_idle)
  Mux : Mux  Inputs=2
  Switch2 : Switch  Threshold=0.5  SaturateOnIntegerOverflow=on  InputSameDT=on
  P_CE : Outport  InitialOutput=0
  wires:
  Constant3/1 -> Switch2/1
  Switch2/1 -> P_CE/1
  P_CE_fuel/1 -> Switch2/3
  Idle detection/1 -> Switch2/2
  w_CE/1 -> Mux/1
  T_CE/1 -> Mux/2
  Mux/1 -> Idle detection/1

== system qss_tb_library/Energy Converter/Combustion Engine (Willans-approximation)/Engine efficiency ==
  w_CE : Inport
  T_CE : Inport  Port=2
  Constant3 : Constant  Value=p_me0g
  Product1 : Product  Inputs=*/  SaturateOnIntegerOverflow=on  RndMeth=Zero  InputSameDT=on
  Sum : Sum  SaturateOnIntegerOverflow=on  InputSameDT=on
  p_me : Fcn  Expr=4*pi*u/V_d
  p_me0 : Sum  SaturateOnIntegerOverflow=on  InputSameDT=on
  p_mef : Fcn  Expr=k1 * (k2 + k3*(S^2)*(u^2)) * PI * sqrt(k4/B)
  p_mf : Fcn  Expr=u/e
  eta_CE : Outport  InitialOutput=0
  wires:
  Product1/1 -> eta_CE/1
  p_me/1 -> Sum/1, Product1/1
  Sum/1 -> p_mf/1
  p_mf/1 -> Product1/2
  p_me0/1 -> Sum/2
  T_CE/1 -> p_me/1
  w_CE/1 -> p_mef/1
  p_mef/1 -> p_me0/1
  Constant3/1 -> p_me0/2

== system qss_tb_library/Energy Converter/Combustion Engine (consumption map)/Detect fuel cutoff ==
  P_CE_fuel : Inport
  T_CE : Inport  Port=2
  Constant1 : Constant  Value=ENABLE_FUEL_CUTOFF
  Constant3 : Constant  Value=P_CE_cutoff
  Decision : Switch  Threshold=0.5
  Detect fuel cutoff : Switch  Threshold=T_CE_cutoff + 0.01  SaturateOnIntegerOverflow=on  InputSameDT=on
  P_CE : Outport
  wires:
  Constant3/1 -> Detect fuel cutoff/3
  T_CE/1 -> Detect fuel cutoff/2
  P_CE_fuel/1 -> Detect fuel cutoff/1, Decision/3
  Detect fuel cutoff/1 -> Decision/1
  Constant1/1 -> Decision/2
  Decision/1 -> P_CE/1

== system qss_tb_library/Energy Converter/Combustion Engine (consumption map)/Detect idle ==
  P_CE_fuel : Inport
  w_CE : Inport  Port=2
  T_CE : Inport  Port=3
  Constant3 : Constant  Value=P_CE_idle
  Idle detection : Fcn  Expr=(u(1) <= w_CE_idle) * (u(2) <= T_CE_idle)
  Mux : Mux  Inputs=2
  Switch2 : Switch  Threshold=0.5  SaturateOnIntegerOverflow=on  InputSameDT=on
  P_CE : Outport  InitialOutput=0
  wires:
  Mux/1 -> Idle detection/1
  T_CE/1 -> Mux/2
  w_CE/1 -> Mux/1
  Idle detection/1 -> Switch2/2
  P_CE_fuel/1 -> Switch2/3
  Switch2/1 -> P_CE/1
  Constant3/1 -> Switch2/1

== system qss_tb_library/Energy Converter/Combustion Engine (consumption map)/Detect overload and overspeed ==
  w_CE : Inport
  T_CE : Inport  Port=2
  Abs : Abs  SaturateOnIntegerOverflow=on
  Constant : Constant  Value=w_CE_upper
  Maximum torque : Lookup  InputValues=w_CE_max  OutputValues=T_CE_max  SaturateOnIntegerOverflow=on
  Saturation : Saturate  UpperLimit=0  LowerLimit=-inf
  Saturation1 : Saturate  UpperLimit=0  LowerLimit=-inf
  Stop Simulation : Stop
  Stop Simulation1 : Stop
  Sum : Sum  Inputs=+-  SaturateOnIntegerOverflow=on  InputSameDT=on
  Sum1 : Sum  Inputs=+-  SaturateOnIntegerOverflow=on  InputSameDT=on
  wires:
  Sum/1 -> Saturation/1
  w_CE/1 -> Maximum torque/1, Sum1/2
  T_CE/1 -> Abs/1
  Maximum torque/1 -> Sum/1
  Abs/1 -> Sum/2
  Saturation/1 -> Stop Simulation/1
  Constant/1 -> Sum1/1
  Sum1/1 -> Saturation1/1
  Saturation1/1 -> Stop Simulation1/1

== system qss_tb_library/Energy Converter/Electric Generator/Detect overload and overspeed ==
  w_EG : Inport
  T_EG : Inport  Port=2
  Abs : Abs  SaturateOnIntegerOverflow=on
  Constant : Constant  Value=w_EG_upper
  Maximum torque : Lookup  InputValues=w_EG_row  OutputValues=T_EG_max  SaturateOnIntegerOverflow=on
  Saturation : Saturate  UpperLimit=0  LowerLimit=-inf
  Saturation1 : Saturate  UpperLimit=0  LowerLimit=-inf
  Stop Simulation : Stop
  Stop Simulation1 : Stop
  Sum : Sum  Inputs=+-  SaturateOnIntegerOverflow=on  InputSameDT=on
  Sum1 : Sum  Inputs=+-  SaturateOnIntegerOverflow=on  InputSameDT=on
  wires:
  Sum/1 -> Saturation/1
  w_EG/1 -> Maximum torque/1, Sum1/2
  T_EG/1 -> Abs/1
  Maximum torque/1 -> Sum/1
  Abs/1 -> Sum/2
  Saturation/1 -> Stop Simulation/1
  Constant/1 -> Sum1/1
  Sum1/1 -> Saturation1/1
  Saturation1/1 -> Stop Simulation1/1

== system qss_tb_library/Energy Converter/Electric Motor/Detect overload and overspeed ==
  w_EM : Inport
  T_EM : Inport  Port=2
  Abs : Abs  SaturateOnIntegerOverflow=on
  Constant : Constant  Value=w_EM_upper
  Maximum torque : Lookup  InputValues=w_EM_row  OutputValues=T_EM_max  SaturateOnIntegerOverflow=on
  Saturation : Saturate  UpperLimit=0  LowerLimit=-inf
  Saturation1 : Saturate  UpperLimit=0  LowerLimit=-inf
  Stop Simulation : Stop
  Stop Simulation1 : Stop
  Sum : Sum  Inputs=+-  SaturateOnIntegerOverflow=on  InputSameDT=on
  Sum1 : Sum  Inputs=+-  SaturateOnIntegerOverflow=on  InputSameDT=on
  wires:
  Saturation1/1 -> Stop Simulation1/1
  Sum1/1 -> Saturation1/1
  Constant/1 -> Sum1/1
  Saturation/1 -> Stop Simulation/1
  Abs/1 -> Sum/2
  Maximum torque/1 -> Sum/1
  T_EM/1 -> Abs/1
  w_EM/1 -> Sum1/2, Maximum torque/1
  Sum/1 -> Saturation/1

== system qss_tb_library/Energy Converter/Fuel Cell/Compressor with E-motor ==
  note: Air mass flow
  P_FC : Inport  Orientation=left
  1/2 O2 for 1 H2 : Gain  Orientation=left  Gain=1/2  SaturateOnIntegerOverflow=on
  Air enthalpy : Gain  Orientation=left  Gain=delta_h_C_air  SaturateOnIntegerOverflow=on
  Air to fuel ratio : Gain  Orientation=left  Gain=l_air  SaturateOnIntegerOverflow=on
  E-motor efficiency : Gain  Orientation=left  Gain=1/eta_EM_C  SaturateOnIntegerOverflow=on
  Inverse O2  fraction : Gain  Orientation=left  Gain=100/21  SaturateOnIntegerOverflow=on
  Lower heating value : Gain  Orientation=left  Gain=1/H_o_m  SaturateOnIntegerOverflow=on
  Molecular weight : Gain  Orientation=left  Gain=M_air  SaturateOnIntegerOverflow=on
  To Workspace4 : ToWorkspace  VariableName=P_EM_C  SampleTime=1  SaveFormat=Array
  Unit Delay : UnitDelay  Orientation=left  SampleTime=h
  P_EM_C : Outport  Orientation=left  InitialOutput=0
  wires:
  Air enthalpy/1 -> E-motor efficiency/1
  Air to fuel ratio/1 -> Air enthalpy/1
  Unit Delay/1 -> Lower heating value/1
  Molecular weight/1 -> Air to fuel ratio/1
  Lower heating value/1 -> 1/2 O2 for 1 H2/1
  1/2 O2 for 1 H2/1 -> Inverse O2  fraction/1
  Inverse O2  fraction/1 -> Molecular weight/1
  E-motor efficiency/1 -> P_EM_C/1, To Workspace4/1
  P_FC/1 -> Unit Delay/1
